simulink model "matrixFtse"  (Simulink 7.3)
settings: Solver=FixedStepDiscrete  StartTime=0.0  StopTime=1070  RelTol=1e-3
PreLoadFcn:
  | [FTSEdata,txt]=xlsread('ftseTrack.xls');
libraries: dspbuff3 x2, dspindex x1, dspsolvers x1, dspsrcs4 x1, dspsnks4 x1
settings Model: Creator=kassama  LastModifiedBy=kassama
settings OptimizationCC: InitFltsAndDblsToZero=on

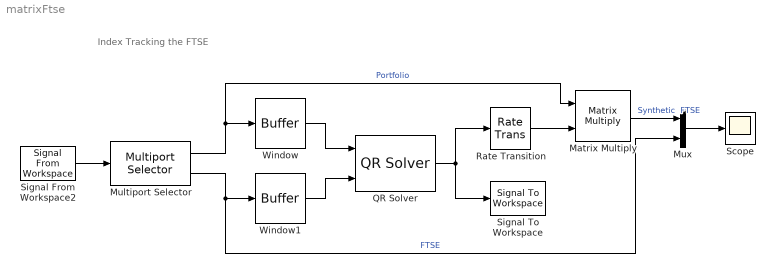
== system matrixFtse ==
  note: Index Tracking the FTSE
  Matrix Multiply : Product  Multiplication=Matrix(*)  OutDataType=sfix(16)  OutScaling=2^0
  Multiport Selector : dspindex/Multiport Selector  rowsOrCols=Columns  idxCellArray={ 3:36,2 }  idxErrMode=Clip Index
  Mux : Mux  Inputs=2
  QR Solver : dspsolvers/QR Solver
  Rate Transition : RateTransition
  Scope : Scope
      settings: YMin=3000  YMax=8000
  Signal From Workspace2 : dspsrcs4/Signal From Workspace  SystemSampleTime=-1  X=FTSEdata  Ts=1  nsamps=1  OutputAfterFinalValue=Setting to zero  ignoreOrWarnInputAndFrameLengths=off
  Signal To Workspace : dspsnks4/Signal To Workspace  SystemSampleTime=-1  VariableName=wts  FrameMode=Concatenate frames (2-D array)
      settings: FixptAsFi=off
  Window : dspbuff3/Buffer  N=100  V=90  ic=0
  Window1 : dspbuff3/Buffer  N=100  V=90  ic=0
  wires:
  Window/1 -> QR Solver/1
  Window1/1 -> QR Solver/2
  QR Solver/1 -> Signal To Workspace/1, Rate Transition/1
  Matrix Multiply/1 -> Mux/1  "Synthetic  FTSE"
  Rate Transition/1 -> Matrix Multiply/2
  Mux/1 -> Scope/1
  Signal From Workspace2/1 -> Multiport Selector/1
  Multiport Selector/1 -> Window/1, Matrix Multiply/1  "Portfolio"
  Multiport Selector/2 -> Window1/1, Mux/2  "FTSE"
